simulink model "gm_ADC_RAW_TO_VALUE"  (R2018a)
settings: Solver=FixedStepDiscrete  StartTime=0.0  StopTime=SimulationsDauer  RelTol=1e-3  EnableMultiTasking=on
undefined symbols (not defined in the file or in its folder): ADC_SET_USER_OFFSET, T_mech
settings Model: Creator=zedboard  LastModifiedBy=Wendel
settings OptimizationCC: BlockReduction=off  ConditionallyExecuteInputs=off  DefaultParameterBehavior=Inlined  LifeSpan=inf
settings DebuggingCC: AlgebraicLoopMsg=error  InheritedTsInSrcMsg=none  SFUnexpectedBacktrackingDiag=warning  SFNoUnconditionalDefaultTransitionDiag=warning  SFExecutionAtInitializationDiag=none
settings HardwareCC: ProdBitPerPointer=32  ProdBitPerSizeT=32  ProdBitPerPtrDiffT=32  ProdLargestAtomicFloat=None  ProdIntDivRoundTo=Undefined  ProdEndianess=Unspecified  ProdWordSize=32  ProdHWDeviceType=ASIC/FPGA->ASIC/FPGA  ProdEqTarget=off
settings CodeAppCC: StateflowObjectComments=on
settings GRTTargetCC: TargetLangStandard=C89/C90 (ANSI)  GeneratePreprocessorConditionals=Disable all
settings ConfigComp: CovMetricSettings=dw  CovHtmlReporting=on  CovSaveCumulativeToWorkspaceVar=on  CovSaveSingleToWorkspaceVar=on  CovExternalEMLEnable=off

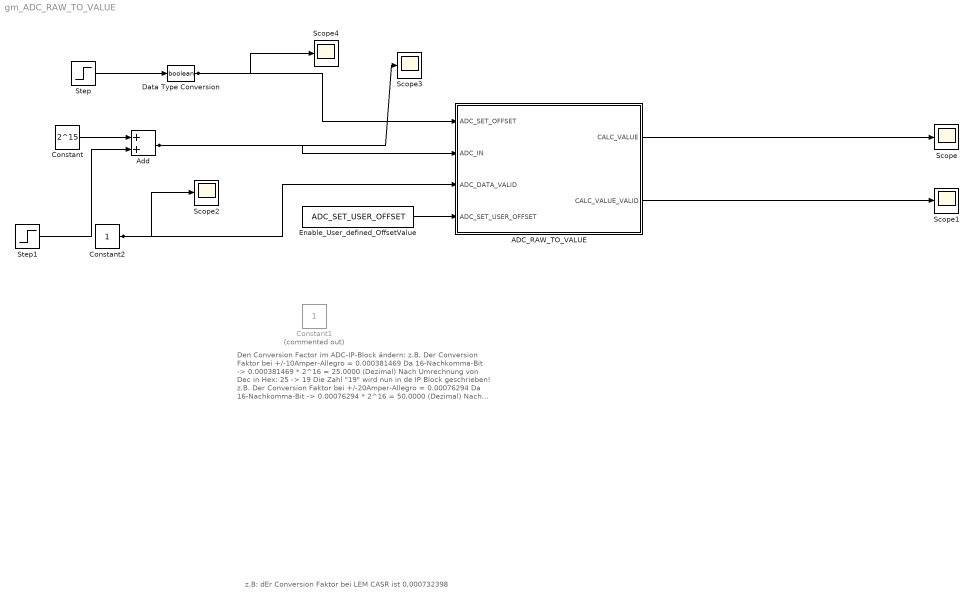
== system gm_ADC_RAW_TO_VALUE ==
  note: Den Conversion Factor im ADC-IP-Block ändern:
      |
      | z.B. Der Conversion Faktor bei +/-10Amper-Allegro = 0.000381469
      | Da 16-Nachkomma-Bit -> 0.000381469 * 2^16 = 25.0000 (Dezimal)
      | Nach Umrechnung von Dec in Hex: 25 -> 19
      | Die Zahl "19" wird nun in de IP Block geschrieben!
      |
      | z.B. Der Conversion Faktor bei +/-20Amper-Allegro = 0.00076294
      | Da 16-Nachkomma-Bit -> 0.00076294 * 2^16 = 50.0000 (Dezimal)
      | Nach Umrechnung von Dec in Hex: 50 -> 32
      | Die Zahl "32" wird nun in de IP Block geschrieben!
      |
      |
      | z.B. Der Conversion Faktor bei Chile Stromsensor = 0.00041018
      | Da 16-Nachkomma-Bit -> 0.00041018 * 2^16 = 26.8816 (Dezimal)
      | Nach Umrechnung von Dec in Hex:  27 -> 1B
      | Die Zahl "1B" wird nun in de IP Block geschrieben!
  note: z.B: dEr Conversion Faktor bei LEM CASR ist 0,000732398
  ADC_RAW_TO_VALUE : Subsystem
  Add : Sum  OutDataTypeStr=Inherit: Same as first input
  Constant : Constant  Value=2^15  OutDataTypeStr=fixdt(0,16,0)  SampleTime=T_mech
  Constant1 : Constant  Commented=on  OutDataTypeStr=boolean
  Constant2 : Constant  OutDataTypeStr=boolean  SampleTime=T_mech
  Data Type Conversion : DataTypeConversion  OutDataTypeStr=boolean
  Enable_User_defined_OffsetValue : Constant  Value=ADC_SET_USER_OFFSET  OutDataTypeStr=boolean  SampleTime=T_mech
  Scope{,1..4} (5 alike) : Scope
  Step : Step  Time=0.01  Before=1  After=0  SampleTime=T_mech
  Step1 : Step  Time=0.02  After=50  SampleTime=T_mech
  wires:
  Enable_User_defined_OffsetValue/1 -> ADC_RAW_TO_VALUE/4(ADC_SET_USER_OFFSET)
  Data Type Conversion/1 -> ADC_RAW_TO_VALUE/1(ADC_SET_OFFSET), Scope4/1
  Step1/1 -> Add/2
  Constant/1 -> Add/1
  ADC_RAW_TO_VALUE/2(CALC_VALUE_VALID) -> Scope1/1
  Constant2/1 -> ADC_RAW_TO_VALUE/3(ADC_DATA_VALID), Scope2/1
  Add/1 -> ADC_RAW_TO_VALUE/2(ADC_IN), Scope3/1
  Step/1 -> Data Type Conversion/1
  ADC_RAW_TO_VALUE/1(CALC_VALUE) -> Scope/1

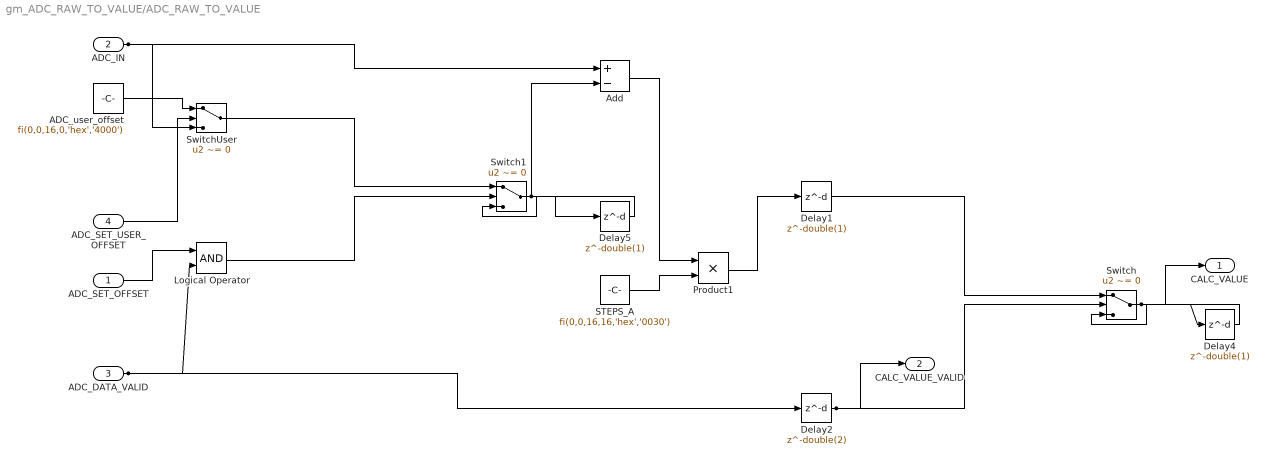
== system gm_ADC_RAW_TO_VALUE/ADC_RAW_TO_VALUE ==
  ADC_SET_OFFSET : Inport  OutDataTypeStr=boolean  PortDimensions=1  SampleTime=1e-07
  ADC_IN : Inport  Port=2  OutDataTypeStr=uint16  PortDimensions=1  SampleTime=1e-07
  ADC_DATA_VALID : Inport  Port=3  OutDataTypeStr=boolean  PortDimensions=1  SampleTime=1e-07
  ADC_SET_USER_OFFSET : Inport  Port=4  OutDataTypeStr=boolean  PortDimensions=1  SampleTime=1e-07
  ADC_user_offset : Constant  Value=fi(0,0,16,0,'hex','4000')  OutDataTypeStr=uint16  SampleTime=-1
  Add : Sum  Inputs=+-  AccumDataTypeStr=fixdt(1, 18, 0)  OutDataTypeStr=fixdt(1, 18, 0)  SampleTime=1e-07
  Delay1 : Delay  DelayLength=double(1)  InitialCondition=0  InputProcessing=Inherited  SampleTime=1e-07
  Delay2 : Delay  DelayLength=double(2)  InitialCondition=0  InputProcessing=Inherited  SampleTime=1e-07
  Delay4 : Delay  DelayLength=double(1)  InitialCondition=0  InputProcessing=Inherited  SampleTime=1e-07
  Delay5 : Delay  DelayLength=double(1)  InitialCondition=0  InputProcessing=Inherited  SampleTime=1e-07
  Logical Operator : Logic  AllPortsSameDT=off  OutDataTypeStr=boolean  SampleTime=1e-07
  Product1 : Product  Inputs=**  OutDataTypeStr=fixdt(1, 18, 11)  SampleTime=1e-07
  STEPS_A : Constant  Value=fi(0,0,16,16,'hex','0030')  OutDataTypeStr=fixdt(0, 16, 16)  SampleTime=-1
  Switch : Switch  Criteria=u2 ~= 0  Threshold=double(0)  OutDataTypeStr=fixdt(1, 18, 11)  SampleTime=1e-07
  Switch1 : Switch  Criteria=u2 ~= 0  Threshold=double(0)  OutDataTypeStr=uint16  SampleTime=1e-07
  SwitchUser : Switch  Criteria=u2 ~= 0  Threshold=double(0)  OutDataTypeStr=uint16  SampleTime=1e-07
  CALC_VALUE : Outport
  CALC_VALUE_VALID : Outport  Port=2
  wires:
  ADC_SET_OFFSET/1 -> Logical Operator/1
  ADC_IN/1 -> SwitchUser/3, Add/1
  ADC_DATA_VALID/1 -> Logical Operator/2, Delay2/1
  ADC_SET_USER_OFFSET/1 -> SwitchUser/2
  ADC_user_offset/1 -> SwitchUser/1
  Add/1 -> Product1/1
  Delay1/1 -> Switch/1
  Delay2/1 -> Switch/2, CALC_VALUE_VALID/1
  Delay4/1 -> Switch/3
  Delay5/1 -> Switch1/3
  Logical Operator/1 -> Switch1/2
  Product1/1 -> Delay1/1
  STEPS_A/1 -> Product1/2
  Switch/1 -> Delay4/1, CALC_VALUE/1
  Switch1/1 -> Add/2, Delay5/1
  SwitchUser/1 -> Switch1/1
